simulink model "AMR_ManualModeControlUnit_24a"  (R2024a)
settings: configuration reference "SharedConfig" (kept outside this file)
undefined symbols (not defined in the file): joy_boost_speed_multiplier, joy_max_speed_multiplier, joy_max_steering_angle, joy_speed
libraries: simulink_extras x1
settings Model: DataDictionary=configuration_dictionary.sldd  Creator=matlab.cut  LastModifiedBy=matlab.cut
settings ConfigSetRef: SourceName=SharedConfig

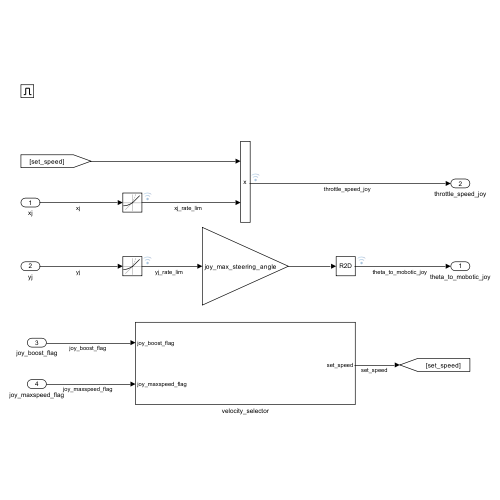
[thumbnail: Simulink's stored preview of the top-level diagram]
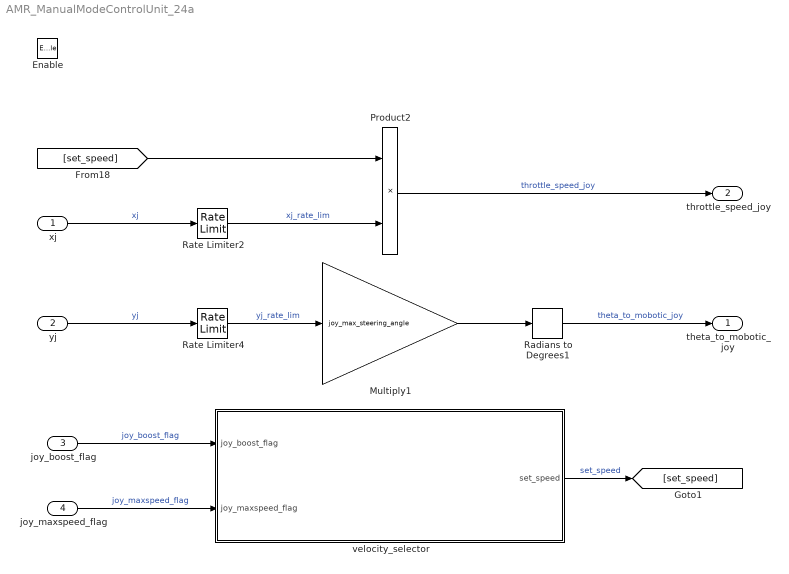
== system AMR_ManualModeControlUnit_24a ==
  xj : Inport
  yj : Inport  Port=2
  joy_boost_flag : Inport  Port=3
  joy_maxspeed_flag : Inport  Port=4
  Enable : EnablePort  OutDataTypeStr=boolean
  Multiply1 : Gain  Gain=joy_max_steering_angle
  Product2 : Product
  Radians to Degrees1 : simulink_extras/Transformations/Radians to Degrees
  Rate Limiter2 : RateLimiter  SampleTimeMode=inherited
  Rate Limiter4 : RateLimiter  RisingSlewLimit=0.5  FallingSlewLimit=-0.5  SampleTimeMode=inherited
  velocity_selector : Subsystem
  theta_to_mobotic_joy : Outport  OutputWhenDisabled=reset  InitialOutput=[0]
  throttle_speed_joy : Outport  Port=2  OutputWhenDisabled=reset  InitialOutput=[0]
  wires:
  yj/1 -> Rate Limiter4/1  "yj"
  Rate Limiter2/1 -> Product2/2  "xj_rate_lim"
  Product2/1 -> throttle_speed_joy/1  "throttle_speed_joy"
  [set_speed] -> Product2/1
  Rate Limiter4/1 -> Multiply1/1  "yj_rate_lim"
  xj/1 -> Rate Limiter2/1  "xj"
  Radians to Degrees1/1 -> theta_to_mobotic_joy/1  "theta_to_mobotic_joy"
  Multiply1/1 -> Radians to Degrees1/1
  velocity_selector/1(set_speed) -> [set_speed]  "set_speed"
  joy_boost_flag/1 -> velocity_selector/1(joy_boost_flag)  "joy_boost_flag"
  joy_maxspeed_flag/1 -> velocity_selector/2(joy_maxspeed_flag)  "joy_maxspeed_flag"

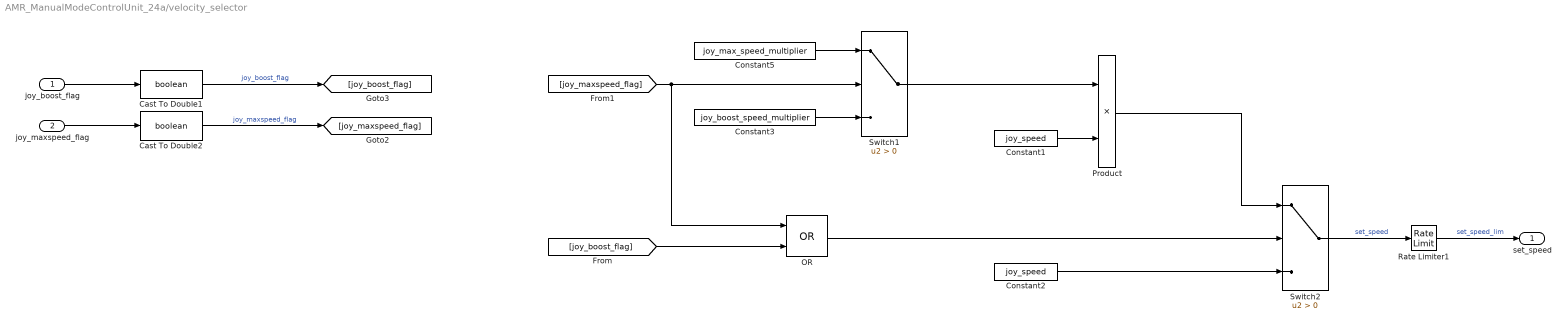
== system AMR_ManualModeControlUnit_24a/velocity_selector ==
  joy_boost_flag : Inport
  joy_maxspeed_flag : Inport  Port=2
  Cast To Double1 : DataTypeConversion  OutDataTypeStr=boolean  SaturateOnIntegerOverflow=off  RndMeth=Floor
  Cast To Double2 : DataTypeConversion  OutDataTypeStr=boolean  SaturateOnIntegerOverflow=off  RndMeth=Floor
  Constant1 : Constant  Value=joy_speed
  Constant2 : Constant  Value=joy_speed
  Constant3 : Constant  Value=joy_boost_speed_multiplier
  Constant5 : Constant  Value=joy_max_speed_multiplier
  OR : Logic  Operator=OR  AllPortsSameDT=off  OutDataTypeStr=boolean
  Product : Product
  Rate Limiter1 : RateLimiter  RisingSlewLimit=300  FallingSlewLimit=-1000  SampleTimeMode=inherited
  Switch1 : Switch  Criteria=u2 > Threshold  SaturateOnIntegerOverflow=off  InputSameDT=off
  Switch2 : Switch  Criteria=u2 > Threshold  SaturateOnIntegerOverflow=off  InputSameDT=off
  set_speed : Outport
  wires:
  Cast To Double2/1 -> [joy_maxspeed_flag]  "joy_maxspeed_flag"
  Cast To Double1/1 -> [joy_boost_flag]  "joy_boost_flag"
  joy_boost_flag/1 -> Cast To Double1/1
  joy_maxspeed_flag/1 -> Cast To Double2/1
  [joy_boost_flag] -> OR/2
  Switch2/1 -> Rate Limiter1/1  "set_speed"
  [joy_maxspeed_flag] -> Switch1/2, OR/1
  Constant3/1 -> Switch1/3
  Constant1/1 -> Product/2
  Constant5/1 -> Switch1/1
  Constant2/1 -> Switch2/3
  OR/1 -> Switch2/2
  Switch1/1 -> Product/1
  Product/1 -> Switch2/1
  Rate Limiter1/1 -> set_speed/1  "set_speed_lim"
